simulink model "DynamicsSim"  (R2016b)
settings: Solver=VariableStepAuto  StartTime=0.0  StopTime=50.0  MaxStep=0.02  RelTol=1e-3
undefined symbols (not defined in the file or in its folder): DrawPlane, GetForces, P
libraries: simulink x3
settings Model: Creator=CFRPG  LastModifiedBy=CFRPG

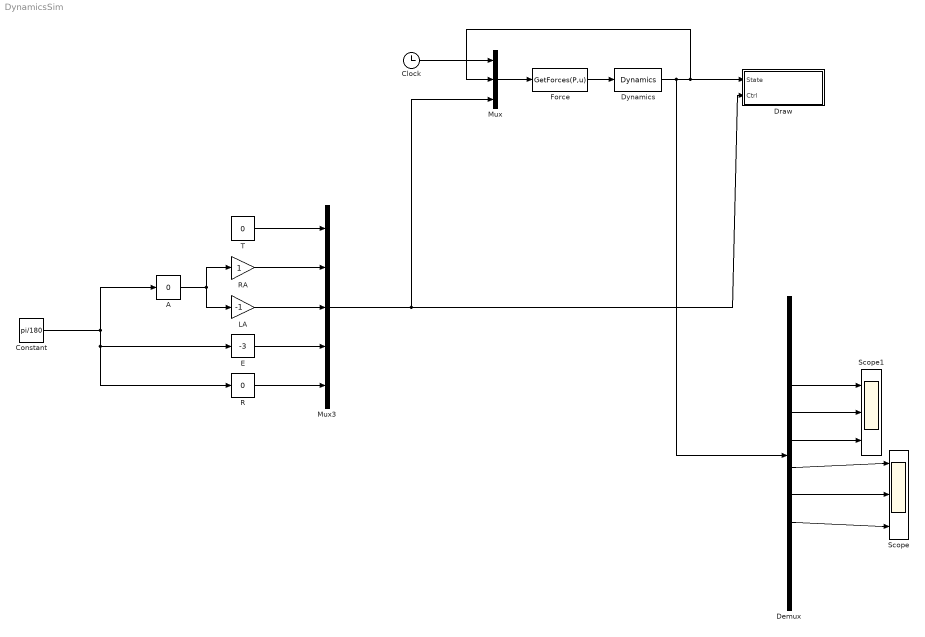
== system DynamicsSim ==
  A : simulink/Math Operations/Slider Gain  low=-360  gain=0  high=360
  Clock : Clock
  Constant : Constant  Value=pi/180
  Demux : Demux  Outputs=12
  Draw : Subsystem
  Dynamics : S-Function  FunctionName=Dynamics  Parameters=P  SFunctionDeploymentMode=off  EnableBusSupport=off
  E : simulink/Math Operations/Slider Gain  low=-360  gain=-3  high=360
  Force : MATLABFcn  MATLABFcn=GetForces(P,u)
  LA : Gain  Gain=-1
  Mux : Mux  Inputs=3
  Mux3 : Mux  Inputs=5
  R : simulink/Math Operations/Slider Gain  low=-360  gain=0  high=360
  RA : Gain
  Scope : Scope  NumInputPorts=3
  Scope1 : Scope  NumInputPorts=3
  T : Constant  Value=0
  wires:
  Dynamics/1 -> Demux/1, Mux/2, Draw/1(State)
  Force/1 -> Dynamics/1
  Mux/1 -> Force/1
  Clock/1 -> Mux/1
  R/1 -> Mux3/5
  E/1 -> Mux3/4
  T/1 -> Mux3/1
  Mux3/1 -> Draw/2(Ctrl), Mux/3
  RA/1 -> Mux3/2
  LA/1 -> Mux3/3
  A/1 -> RA/1, LA/1
  Constant/1 -> A/1, E/1, R/1
  Demux/7 -> Scope/1
  Demux/8 -> Scope/2
  Demux/9 -> Scope/3
  Demux/5 -> Scope1/2
  Demux/4 -> Scope1/1
  Demux/6 -> Scope1/3

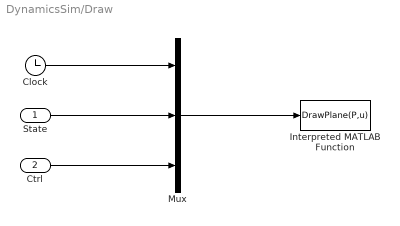
== system DynamicsSim/Draw ==
  State : Inport
  Ctrl : Inport  Port=2
  Clock : Clock
  Interpreted MATLAB Function : MATLABFcn  MATLABFcn=DrawPlane(P,u)  OutputDimensions=0
  Mux : Mux  Inputs=3
  wires:
  State/1 -> Mux/2
  Clock/1 -> Mux/1
  Ctrl/1 -> Mux/3
  Mux/1 -> Interpreted MATLAB Function/1
